simulink model "q2_b_simulink_PD"  (R2013a)
settings: Solver=ode45  StartTime=0.0  StopTime=3  RelTol=1e-3
values from neighbouring files (symbols this model uses):
  Kd = Kd_temp    [f.m]    (also in q2_b_PD.m = x1)
  Kp = Kp_temp    [f.m]    (also in q2_b_PD.m = x2)
settings Model: Creator=obrien94  LastModifiedBy=obrien94

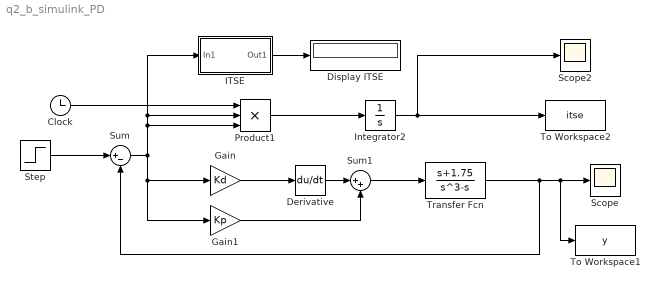
== system q2_b_simulink_PD ==
  Clock : Clock
  Derivative : Derivative
  Display ITSE : Display
  Gain : Gain  Gain=Kd
  Gain1 : Gain  Gain=Kp
  ITSE : Subsystem
      mask help:
      | ISE performance index
      |
      | output = int (input)^2 dt
      mask Display:
      | disp('ITSE')
      | port_label('input',1,'e')
      | port_label('output',1,'itse')
  Integrator2 : Integrator
  Product1 : Product  Inputs=3
  Scope : Scope
  Scope2 : Scope
      settings: SaveName=ScopeData2
  Step : Step  SampleTime=0
  Sum : Sum  Inputs=|+-
  Sum1 : Sum  Inputs=|++
  To Workspace1 : ToWorkspace  VariableName=y  SampleTime=-1  SaveFormat=Timeseries
  To Workspace2 : ToWorkspace  VariableName=itse  SampleTime=-1
  Transfer Fcn : TransferFcn  Numerator=[1 1.75]  Denominator=[1 0 -1 0]
  wires:
  Step/1 -> Sum/1
  Sum/1 -> Gain/1, Gain1/1, Product1/3, Product1/2, ITSE/1(In1)
  Transfer Fcn/1 -> Sum/2, To Workspace1/1, Scope/1
  Gain/1 -> Derivative/1
  Derivative/1 -> Sum1/1
  Sum1/1 -> Transfer Fcn/1
  Gain1/1 -> Sum1/2
  Integrator2/1 -> Scope2/1, To Workspace2/1
  Product1/1 -> Integrator2/1
  Clock/1 -> Product1/1
  ITSE/1(Out1) -> Display ITSE/1

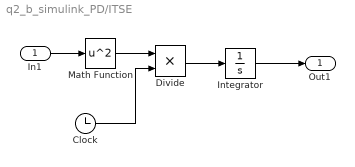
== system q2_b_simulink_PD/ITSE ==
  In1 : Inport
  Clock : Clock
  Divide : Product  Inputs=**
  Integrator : Integrator
  Math Function : Math  Operator=square  SaturateOnIntegerOverflow=on
  Out1 : Outport
  wires:
  Integrator/1 -> Out1/1
  In1/1 -> Math Function/1
  Divide/1 -> Integrator/1
  Math Function/1 -> Divide/1
  Clock/1 -> Divide/2
